simulink model "simulateur"  (R2023b)
settings: Solver=VariableStepAuto  StartTime=0.0  StopTime=50  RelTol=1e-3
settings Model: Creator=Morin  LastModifiedBy=haoyuan
settings SolverCC: AlgebraicLoopSolver=TrustRegion
settings DebuggingCC: UnconnectedInputMsg=warning  UnconnectedOutputMsg=warning  UnconnectedLineMsg=warning
settings ModelReferenceCC: EnableRefExpFcnMdlSchedulingChecks=on

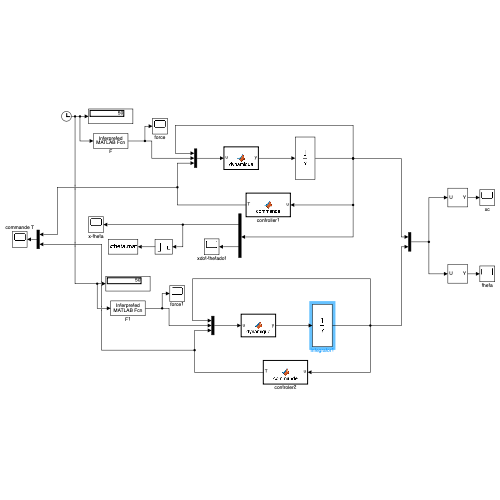
[thumbnail: Simulink's stored preview of the top-level diagram]
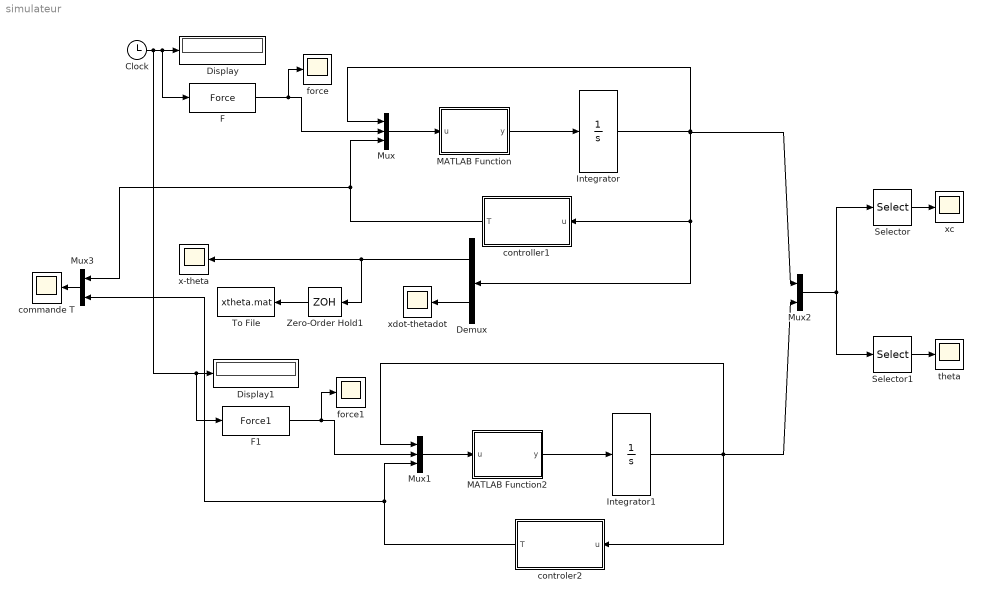
== system simulateur ==
  Clock : Clock
  Demux : Demux  Outputs=2
  Display : Display
  Display1 : Display
  F : MATLABFcn  MATLABFcn=Force  OutputDimensions=1
  F1 : MATLABFcn  MATLABFcn=Force1  OutputDimensions=1
  Integrator : Integrator  InitialCondition=[0.1;0;1e-8;0]
  Integrator1 : Integrator  InitialCondition=[0.1;0;1e-8;0]
  MATLAB Function : MATLAB Function  TreatAsAtomicUnit=on
  MATLAB Function2 : MATLAB Function  TreatAsAtomicUnit=on
  Mux : Mux  Inputs=3
  Mux1 : Mux  Inputs=3
  Mux2 : Mux  Inputs=2
  Mux3 : Mux  Inputs=2
  Selector : Selector  InputPortWidth=8  IndexOptions=Index vector (dialog)  Indices=[1 5]  OutputSizes=1
  Selector1 : Selector  InputPortWidth=8  IndexOptions=Index vector (dialog)  Indices=[3 7]  OutputSizes=1
  To File : ToFile  Filename=xtheta.mat  SaveFormat=Timeseries  SampleTime=0.01
  Zero-Order Hold1 : ZeroOrderHold  SampleTime=0.01
  commande T : Scope
  controler2 : MATLAB Function  TreatAsAtomicUnit=on
  controller1 : MATLAB Function  TreatAsAtomicUnit=on
  force : Scope
  force1 : Scope
  theta : Scope
  x-theta : Scope
  xc : Scope
  xdot-thetadot : Scope
  wires:
  MATLAB Function/1(y) -> Integrator/1
  Integrator/1 -> Demux/1, controller1/1(u), Mux2/1, Mux/1
  Mux/1 -> MATLAB Function/1(u)
  Demux/1 -> Zero-Order Hold1/1, x-theta/1
  Demux/2 -> xdot-thetadot/1
  controller1/1(T) -> Mux/3, Mux3/1
  Zero-Order Hold1/1 -> To File/1
  F/1 -> force/1, Mux/2
  controler2/1(T) -> Mux3/2, Mux1/3
  Mux1/1 -> MATLAB Function2/1(u)
  MATLAB Function2/1(y) -> Integrator1/1
  Integrator1/1 -> Mux1/1, Mux2/2, controler2/1(u)
  Clock/1 -> F1/1, Display1/1, F/1, Display/1
  F1/1 -> force1/1, Mux1/2
  Mux2/1 -> Selector1/1, Selector/1
  Selector/1 -> xc/1
  Selector1/1 -> theta/1
  Mux3/1 -> commande T/1

== matlab function simulateur/MATLAB Function ==
  data: u input; y output
function y = dynamique(u)
% fonction définissant la dynamique du système: renvoie f(X,U) avec X
% l'état, et U la variable de commande physique (composante T de la force
% appliquée au chariot)

x= u(1); %position du chariot
xdot= u(2); %inclinaison de la barre
theta= u(3); % vitesse du chariot
thetadot= u(4); % vitesse angulaire de la barre
F=u(5);
T= u(6); % force appliquée au chariot

% Defintion des paramètres du système
m= 0.2; % masse de la barre
M= 1; % masse chario
l= 0.2; % demi-longueur de la barre
J=  m*l^2/3; % inertie de la barre
g= 9.81; % cste de gravité
k=180; %raideur de ressort
%mu= 0.005; % coeff. de frottement visqueux barre
%tau= 0.2; % coeff. de frottement visqueux chariot

%defini les changement de varriable 

xd=sqrt((M+m)/(J+m*l^2))*x;
xd_dot=sqrt((M+m)/(J+m*l^2))*xdot;
eps=m*l/(sqrt((J+m*l^2)*(M+m)));   
u=(M+m)/(k*(J+m*l^2))*(T-m*g*l*sin(theta));
Fd=1/k*sqrt((M+m)/(J+m*l^2))*F;


% defini le modele dynamique
x1=xd;
x2=xd_dot;
x3=theta;
x4=thetadot;

fx=[x2;(-x1+eps*x4^2*sin(x3))/(1-eps^2*cos(x3)^2);x4;eps*cos(x3)*(x1-eps*x4^2*sin(x3))/(1-eps^2*cos(x3)^2)];
gx=1/(1-eps^2*cos(x3)^2)*[0;-eps*cos(x3);0;1];
dx=1/(1-eps^2*cos(x3)^2)*[0;1;0;-eps*cos(x3)];


vector=fx+gx*u+dx*Fd;%xddot xddotdot thetadot thetadotdot
vector(1)=vector(1)*sqrt((J+m*l^2)/(M+m));%xddot->xdot
vector(2)=vector(2)*sqrt((J+m*l^2)/(M+m));%xddotdot->xdotdot


%Calcul de f
y=vector;

== matlab function simulateur/MATLAB Function2 ==
  data: u input; y output
function y = dynamique(u)
% fonction définissant la dynamique du système: renvoie f(X,U) avec X
% l'état, et U la variable de commande physique (composante T de la force
% appliquée au chariot)

x= u(1); %position du chariot
xdot= u(2); %inclinaison de la barre
theta= u(3); % vitesse du chariot
thetadot= u(4); % vitesse angulaire de la barre
F=u(5);
T= u(6); % force appliquée au chariot

% Defintion des paramètres du système
m= 0.2; % masse de la barre
M= 1; % masse chario
l= 0.2; % demi-longueur de la barre
J=  m*l^2/3; % inertie de la barre
g= 9.81; % cste de gravité
k=180; %raideur de ressort
%mu= 0.005; % coeff. de frottement visqueux barre
%tau= 0.2; % coeff. de frottement visqueux chariot

%defini les changement de varriable 

xd=sqrt((M+m)/(J+m*l^2))*x;
xd_dot=sqrt((M+m)/(J+m*l^2))*xdot;
eps=m*l/(sqrt((J+m*l^2)*(M+m)));   
u=(M+m)/(k*(J+m*l^2))*(T-m*g*l*sin(theta));
Fd=1/k*sqrt((M+m)/(J+m*l^2))*F;


% defini le modele dynamique
x1=xd;
x2=xd_dot;
x3=theta;
x4=thetadot;

fx=[x2;(-x1+eps*x4^2*sin(x3))/(1-eps^2*cos(x3)^2);x4;eps*cos(x3)*(x1-eps*x4^2*sin(x3))/(1-eps^2*cos(x3)^2)];
gx=1/(1-eps^2*cos(x3)^2)*[0;-eps*cos(x3);0;1];
dx=1/(1-eps^2*cos(x3)^2)*[0;1;0;-eps*cos(x3)];


vector=fx+gx*u+dx*Fd;%xddot xddotdot thetadot thetadotdot
vector(1)=vector(1)*sqrt((J+m*l^2)/(M+m));%xddot->xdot
vector(2)=vector(2)*sqrt((J+m*l^2)/(M+m));%xddotdot->xdotdot


%Calcul de f
y=vector;

== matlab function simulateur/controler2 ==
  data: u input; T output
function T = commande(u)
% Fonction qui calcule la commande T

% Définition des états
x= u(1);
xdot= u(2);
theta= u(3);
thetadot=u(4);

% Definition des paramètres du système
m= 0.2; % masse de la barre
M= 1; % masse chariot
l= 0.2; % demi-longueur de la barre
J=  m*l^2/3; % inertie de la barre
g= 9.81; % cste de gravité
k=180; %raideur de ressort

%definir changement de varriable 
xd=sqrt((M+m)/(J+m*l^2))*x;
xd_dot=sqrt((M+m)/(J+m*l^2))*xdot;
eps=m*l/(sqrt((J+m*l^2)*(M+m)));   

x1=xd;
x2=xd_dot;
x3=theta;
x4=thetadot;
%definir les parametre de controler

%controler1
p0=1;p1=1;p2=1;c0=1;c1=1;c2=1;
%controler2
%p0=10;p1=0.1;c0=1.9;p2=1;c1=1;c2=1;

%nouvelle varriable
z1=x1+eps*sin(x3);
z2=x2+eps*x4*cos(x3);

%consider the problem of stabilisation with y1 as the control input
k1=-c0*atan(z2);
y1=x3;
k2=-c1*(y1+c0*atan(z2))+c0*(z1-eps*sin(y1))/(1+z2^2)-eps*p0*z2/(p1*(y1+c0*atan(z2)))*(sin(y1)+sin(c0*atan(z2)));
y2=x4;



%%
K1=c0/(1+z2^2);
K2=-eps*p0/(p1*(y1+c0*atan(z2)))*(sin(y1)+sin(c0*atan(z2))+c0*z2*cos(c0*atan(z2))/(1+z2^2))-c0*c1/(1+z2^2)-2*c0*z2*(z1-eps*sin(y1))/(1+z2^2)^2+eps*p0*c0/p1*z2*(sin(y1)+sin(c0*atan(z2)))/((1+z2^2)*(y1+c0*atan(z2))^2);
K3=-c1-eps*c0*cos(y1)/(1+z2^2)-eps*p0/p1*z2*cos(y1)/(y1+c0*atan(z2))+eps*p0/p1*z2*(sin(y1)+sin(c0*atan(z2)))/(y1+c0*atan(z2))^2;

%loi de commande pour le nouveau champs z1 z2 y1 y2
v=-c2*(y2-k2)+K1*z2+K2*(-z1+eps*sin(y1))+K3*y2-p1/p2*(y1+c0*atan(z2));
u=(1-eps^2*cos(x3)^2)*v-eps*x1*cos(x3)+eps^2*x4^2*cos(x3)*sin(x3);
T=u*k*(J+m*l^2)/(M+m)+m*g*l*sin(theta);

== matlab function simulateur/controller1 ==
  data: u input; T output
function T = commande(u)
% Fonction qui calcule la commande T

% Définition des états
x= u(1);
xdot= u(2);
theta= u(3);
thetadot=u(4);

% Definition des paramètres du système
m= 0.2; % masse de la barre
M= 1; % masse chariot
l= 0.2; % demi-longueur de la barre
J=  m*l^2/3; % inertie de la barre
g= 9.81; % cste de gravité
k=180; %raideur de ressort

%definir changement de varriable 
xd=sqrt((M+m)/(J+m*l^2))*x;
xd_dot=sqrt((M+m)/(J+m*l^2))*xdot;
eps=m*l/(sqrt((J+m*l^2)*(M+m)));   

x1=xd;
x2=xd_dot;
x3=theta;
x4=thetadot;
%definir les parametre de controler

%controler1
%p0=1;p1=1;p2=1;c0=1;c1=1;c2=1;
%controler2
p0=10;p1=0.1;c0=1.9;p2=1;c1=1;c2=1;

%nouvelle varriable
z1=x1+eps*sin(x3);
z2=x2+eps*x4*cos(x3);

%consider the problem of stabilisation with y1 as the control input
k1=-c0*atan(z2);
y1=x3;
k2=-c1*(y1+c0*atan(z2))+c0*(z1-eps*sin(y1))/(1+z2^2)-eps*p0*z2/(p1*(y1+c0*atan(z2)))*(sin(y1)+sin(c0*atan(z2)));
y2=x4;



%%
K1=c0/(1+z2^2);
K2=-eps*p0/(p1*(y1+c0*atan(z2)))*(sin(y1)+sin(c0*atan(z2))+c0*z2*cos(c0*atan(z2))/(1+z2^2))-c0*c1/(1+z2^2)-2*c0*z2*(z1-eps*sin(y1))/(1+z2^2)^2+eps*p0*c0/p1*z2*(sin(y1)+sin(c0*atan(z2)))/((1+z2^2)*(y1+c0*atan(z2))^2);
K3=-c1-eps*c0*cos(y1)/(1+z2^2)-eps*p0/p1*z2*cos(y1)/(y1+c0*atan(z2))+eps*p0/p1*z2*(sin(y1)+sin(c0*atan(z2)))/(y1+c0*atan(z2))^2;

%loi de commande pour le nouveau champs z1 z2 y1 y2
v=-c2*(y2-k2)+K1*z2+K2*(-z1+eps*sin(y1))+K3*y2-p1/p2*(y1+c0*atan(z2));
u=(1-eps^2*cos(x3)^2)*v-eps*x1*cos(x3)+eps^2*x4^2*cos(x3)*sin(x3);
T=u*k*(J+m*l^2)/(M+m)+m*g*l*sin(theta);


%T=1;
